simulink model "hwk_1"  (R2021a)
settings: Solver=ode4  StartTime=0.0  StopTime=3  FixedStep=0.01  RelTol=1e-3
values from neighbouring files (symbols this model uses):
  G = nd2sys(1,conv([10 1],conv([0.05 1],[0.05 1])),200)    [hmw1.m]
  G_d = Gd_term*H    [hmw1.m]
  Gd_term = 0.5    [hmw1.m]
  H = tf([200],[10 1])    [hmw1.m]
  K1 = 0.5    [hmw1.m]
  K2 = tf([K1 2*K1],[1 0])    [hmw1.m]
  K3 = K2* tf([0.05 1],[0.005 1])    [hmw1.m]
  Plant = G*H    [hmw1.m]
libraries: pid_lib x1
settings Model: PacingRate=0.100000  Creator=aycak  LastModifiedBy=aycak

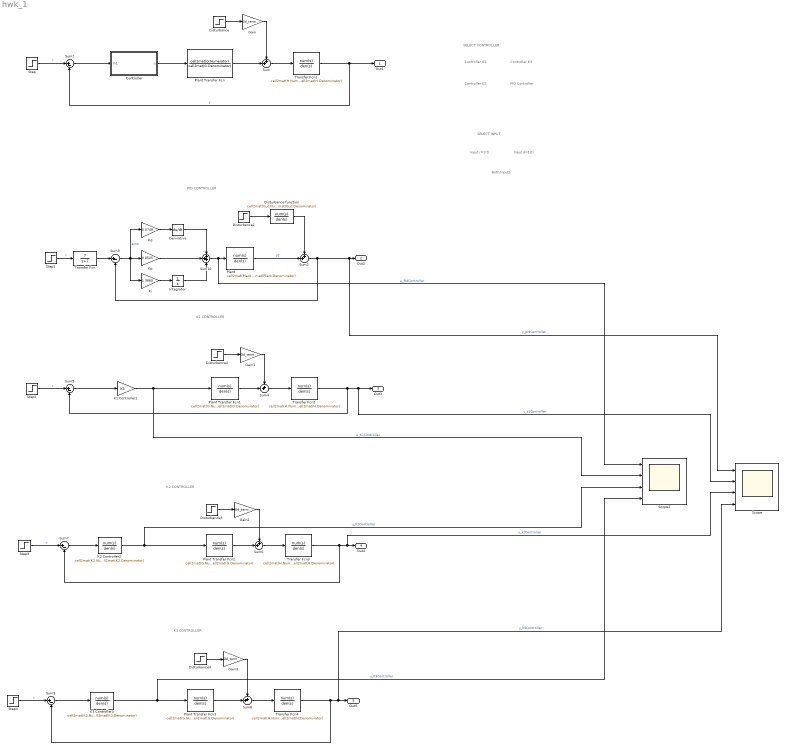
== system hwk_1 ==
  note: PID CONTROLLER
  note: SELECT CONTROLLER
  note: Controller K1
  note: Controller K2
  note: Controller K3
  note: PID Controller
  note: SELECT INPUT
  note: Input r=1(t)
  note: Input d=1(t)
  note: Both Inputs
  note: K1 CONTROLLER
  note: K2 CONTROLLER
  note: K3 CONTROLLER
  Controller : Subsystem
  Derivative : Derivative
  Disturbance : Step  After=0  SampleTime=0
  Disturbance function : TransferFcn  Numerator=cell2mat(G_d.Numerator)  Denominator=cell2mat(G_d.Denominator)
  Disturbance{1..4} (4 alike) : Step  SampleTime=0
  Gain{,1..3} (4 alike) : Gain  Gain=Gd_term
  Integrator : Integrator
  K1 Controller1 : Gain  Gain=K1
  K2 Controller2 : TransferFcn  Numerator=cell2mat(K2.Numerator)  Denominator=cell2mat(K2.Denominator)
  K3 Controller3 : TransferFcn  Numerator=cell2mat(K3.Numerator)  Denominator=cell2mat(K3.Denominator)
  Kd : Gain  Gain=0.0748
  Ki : Gain  Gain=1.3880
  Kp : Gain  Gain=0.8525
  Plant : TransferFcn  Numerator=cell2mat(Plant.Numerator)  Denominator=cell2mat(Plant.Denominator)
  Plant Transfer Fcn{,1..3} (4 alike) : TransferFcn  Numerator=cell2mat(G.Numerator)  Denominator=cell2mat(G.Denominator)
  Scope : Scope  NumInputPorts=4
  Scope2 : Scope  NumInputPorts=4
  Step : Step  SampleTime=0
  Step{1..4} (4 alike) : Step  After=0  SampleTime=0
  Sum{,2,4,6,8} (5 alike) : Sum  Inputs=++|
  Sum{1,3,5,7,9} (5 alike) : Sum  Inputs=|+-
  Sum10 : Sum  Inputs=+++
  Transfer Fcn : TransferFcn  Numerator=[7]  Denominator=[1 7]
  Transfer Fcn{1..4} (4 alike) : TransferFcn  Numerator=cell2mat(H.Numerator)  Denominator=cell2mat(H.Denominator)
  Out1 : Outport  SignalName=yout
  Out2 : Outport  Port=2  SignalName=yout
  Out3 : Outport  Port=3  SignalName=yout
  Out4 : Outport  Port=4  SignalName=yout
  Out5 : Outport  Port=5  SignalName=yout
  wires:
  Sum/1 -> Transfer Fcn1/1
  Plant Transfer Fcn/1 -> Sum/2
  Gain/1 -> Sum/1
  Transfer Fcn1/1 -> Sum1/2, Out1/1  "y"
  Step/1 -> Sum1/1  "r"
  Disturbance/1 -> Gain/1
  Sum2/1 -> Scope/1, Out2/1, Sum3/2  "y_pidController"
  Disturbance function/1 -> Sum2/1
  Disturbance1/1 -> Disturbance function/1
  Sum3/1 -> Kd/1, Kp/1, Ki/1  "error"
  Plant/1 -> Sum2/2  "y2"
  Sum5/1 -> K1 Controller1/1
  Sum4/1 -> Transfer Fcn2/1
  Plant Transfer Fcn1/1 -> Sum4/2
  Disturbance2/1 -> Gain1/1
  Step2/1 -> Sum5/1  "r"
  Transfer Fcn2/1 -> Sum5/2, Scope/2, Out3/1  "y_k1Controller"
  Gain1/1 -> Sum4/1
  Gain2/1 -> Sum6/1
  Transfer Fcn3/1 -> Scope/3, Out4/1, Sum7/2  "y_k2Controller"
  Plant Transfer Fcn2/1 -> Sum6/2
  Disturbance3/1 -> Gain2/1
  Step3/1 -> Sum7/1  "r"
  Sum6/1 -> Transfer Fcn3/1
  K3 Controller3/1 -> Scope2/4, Plant Transfer Fcn3/1  "u_K3Controller"
  Sum9/1 -> K3 Controller3/1
  Sum8/1 -> Transfer Fcn4/1
  Disturbance4/1 -> Gain3/1
  Step4/1 -> Sum9/1  "r"
  Gain3/1 -> Sum8/1
  Transfer Fcn4/1 -> Scope/4, Out5/1, Sum9/2  "y_k3Controller"
  Plant Transfer Fcn3/1 -> Sum8/2
  K2 Controller2/1 -> Scope2/3, Plant Transfer Fcn2/1  "u_K2Controller"
  Sum7/1 -> K2 Controller2/1
  K1 Controller1/1 -> Scope2/2, Plant Transfer Fcn1/1  "u_K1Controller"
  Step1/1 -> Transfer Fcn/1  "r"
  Transfer Fcn/1 -> Sum3/1
  Ki/1 -> Integrator/1
  Integrator/1 -> Sum10/3
  Kd/1 -> Derivative/1
  Derivative/1 -> Sum10/1
  Kp/1 -> Sum10/2
  Sum10/1 -> Scope2/1, Plant/1  "u_PidController"
  Sum1/1 -> Controller/1(In1)
  Controller/1(u) -> Plant Transfer Fcn/1

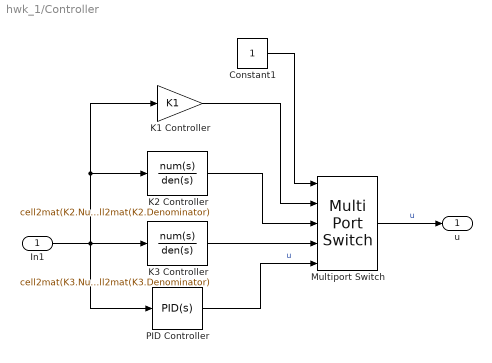
== system hwk_1/Controller ==
  In1 : Inport
  Constant1 : Constant
  K1 Controller : Gain  Gain=K1
  K2 Controller : TransferFcn  Numerator=cell2mat(K2.Numerator)  Denominator=cell2mat(K2.Denominator)
  K3 Controller : TransferFcn  Numerator=cell2mat(K3.Numerator)  Denominator=cell2mat(K3.Denominator)
  Multiport Switch : MultiPortSwitch  Inputs=4
  PID Controller : pid_lib/PID Controller  Controller=PID  Form=Parallel  TimeDomain=Continuous-time  UseExternalTs=off  SampleTime=-1  IntegratorMethod=Forward Euler  FilterMethod=Forward Euler  ControllerParametersSource=internal  P=0  I=0.000195830242380093  D=0  UseFilter=on  N=100  TunerSelectOption=Transfer Function Based (PID Tuner App)  InitialConditionSource=internal  InitialConditionForIntegrator=0  InitialConditionForFilter=0  DifferentiatorICPrevScaledInput=0  ExternalReset=none  TrackingMode=off  Kt=1  LimitOutput=off  SatLimitsSource=internal  UpperSaturationLimit=inf  LowerSaturationLimit=-inf  LinearizeAsGain=on  AntiWindupMode=none  Kb=1  POutMin=[]  POutMax=[]  IOutMin=[]  IOutMax=[]  DOutMin=[]  DOutMax=[]  NOutMin=[]  NOutMax=[]  SumOutMin=[]  SumOutMax=[]  SaturationOutMin=[]  SaturationOutMax=[]  PParamMin=[]  PParamMax=[]  IParamMin=[]  IParamMax=[]  DParamMin=[]  DParamMax=[]  NParamMin=[]  NParamMax=[]  KbParamMin=[]  KbParamMax=[]  KtParamMin=[]  KtParamMax=[]  KbOutMin=[]  KbOutMax=[]  KtOutMin=[]  KtOutMax=[]  IntegratorOutMin=[]  IntegratorOutMax=[]  FilterOutMin=[]  FilterOutMax=[]  SumI1OutMin=[]  SumI1OutMax=[]  SumI2OutMin=[]  SumI2OutMax=[]  SumI3OutMin=[]  SumI3OutMax=[]  SumI4OutMin=[]  SumI4OutMax=[]  SumDOutMin=[]  SumDOutMax=[]  DifferentiatorOutMin=[]  DifferentiatorOutMax=[]  FilterDiffOutCoefMin=[]  FilterDiffOutCoefMax=[]  ReciprocalOutMin=[]  ReciprocalOutMax=[]  SumDenOutMin=[]  SumDenOutMax=[]  SumNumOutMin=[]  SumNumOutMax=[]  DivideOutMin=[]  DivideOutMax=[]  UdiffTsProdOutMin=[]  UdiffTsProdOutMax=[]  NTsProdOutMin=[]  NTsProdOutMax=[]  UintegralTsProdOutMin=[]  UintegralTsProdOutMax=[]  UngainTsProdOutMin=[]  UngainTsProdOutMax=[]  IntegratorContinuousStateAttributes=''  IntegratorStateMustResolveToSignalObject=off  IntegratorRTWStateStorageClass=Auto  FilterContinuousStateAttributes=''  FilterStateMustResolveToSignalObject=off  FilterRTWStateStorageClass=Auto  ParallelPVariant=InternalParameters  IdealPVariant=Disabled  IVariant=InternalParameters  DVariant=InternalParameters  IntegratorVariant=Continuous  SatVariant=Disabled  AWVariant=Passthrough  PCopyVariant=Disabled  TRVariant=Disabled  FdbkBlocksVariant=Forward  IdealPFdbkVariant=Disabled  SatFdbkVariant=Disabled  DerivativeFilterVariant=ContFilter  NVariant=InternalParameters  NCopyVariant=Disabled  FilterICVariant=InternalICsFilter  IntegratorICVariant=InternalICs  ExternalResetVariant=Disabled  TRSumVariant=Passthrough  SumFdbkVariant=Disabled  SumVariant=Sum_PID  TsampFilterVariant=InternalTs  TsampNgainVariant=Passthrough  TsampIntegralVariant=Passthrough  ExternalSaturationOutDataTypeStr=Inherit: Same as second input
  u : Outport
  wires:
  K2 Controller/1 -> Multiport Switch/3
  In1/1 -> K1 Controller/1, K2 Controller/1, K3 Controller/1, PID Controller/1
  K1 Controller/1 -> Multiport Switch/2
  K3 Controller/1 -> Multiport Switch/4
  Constant1/1 -> Multiport Switch/1
  PID Controller/1 -> Multiport Switch/5  "u"
  Multiport Switch/1 -> u/1  "u"
